simulink model "robot_controller"  (R2024a)
settings: Solver=FixedStepDiscrete  StartTime=0.0  StopTime=10.0  FixedStep=0.1  RelTol=1e-3  EnableMultiTasking=on
settings Model: ExtModeTrigDuration=2  Creator=amir  LastModifiedBy=amir
settings SolverCC: AutoInsertRateTranBlk=on  EnableFixedStepZeroCrossing=on
settings OptimizationCC: DefaultParameterBehavior=Inlined  UseDivisionForNetSlopeComputation=on  GainParamInheritBuiltInType=on  UseFloatMulNetSlope=on  InlineInvariantSignals=on  PassReuseOutputArgsAs=Individual arguments  ZeroExternalMemoryAtStartup=off  ZeroInternalMemoryAtStartup=off  NoFixptDivByZeroProtection=on  EfficientFloat2IntCast=on  LifeSpan=1  MaxStackSize=64  OptimizeBlockOrder=speed  DifferentSizesBufferReuse=on  EfficientTunableParamExpr=on
settings DebuggingCC: ParameterTunabilityLossMsg=error
settings HardwareCC: ProdBitPerInt=16  ProdBitPerPointer=16  ProdBitPerSizeT=16  ProdBitPerPtrDiffT=16  ProdLargestAtomicFloat=None  ProdWordSize=8  ProdLongLongMode=on  ProdHWDeviceType=Atmel->AVR
settings SFSimCC: MATLABDynamicMemAlloc=off
settings RTWCC: Description=Embedded Coder  SystemTargetFile=ert.tlc  HardwareBoard=Arduino Uno  TemplateMakefile=ert_default_tmf  Toolchain=Arduino AVR  BuildConfiguration=Faster Runs
settings CodeAppCC: ForceParamTrailComments=on  IgnoreCustomStorageClasses=off  OperatorAnnotations=on  SimulinkDataObjDesc=on  SFDataObjDesc=on  CustomSymbolStrGlobalVar=rt$N$M  CustomSymbolStrType=$N$M  CustomSymbolStrFcn=$N$M$F  CustomSymbolStrMacro=$N$M  InsertBlockDesc=on
settings ERTTargetCC: IncludeMdlTerminateFcn=off  CombineSignalStateStructs=on  SupportAbsoluteTime=off  SupportComplex=off  SupportNonInlinedSFcns=on  ExtModeTransport=3  ExtModeStaticAlloc=on  ExtModeAutomaticAllocSize=off  ExtModeStaticAllocSize=250  ExtModeMexFile=ext_xcp  ExtModeIntrfLevel=Level2 - Open  InlinedParameterPlacement=NonHierarchical  ERTFilePackagingFormat=CompactWithDataFile

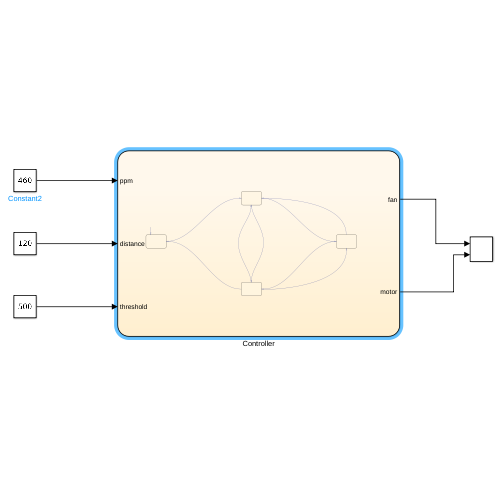
[thumbnail: Simulink's stored preview of the top-level diagram]
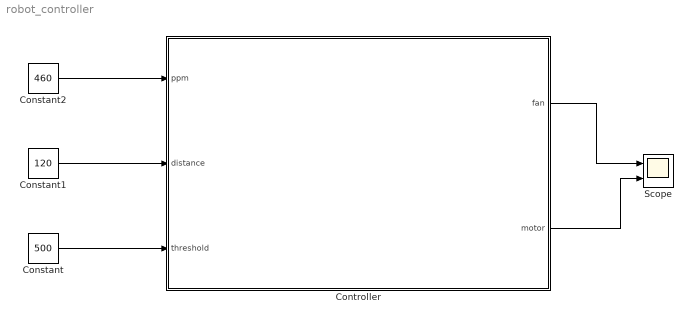
== system robot_controller ==
  Constant : Constant  Value=500
  Constant1 : Constant  Value=120
  Constant2 : Constant  Value=460
  Controller : Stateflow chart  TreatAsAtomicUnit=on
  Scope : Scope  NumInputPorts=2
  wires:
  Controller/1(fan) -> Scope/1
  Controller/2(motor) -> Scope/2
  Constant/1 -> Controller/3(threshold)
  Constant1/1 -> Controller/2(distance)
  Constant2/1 -> Controller/1(ppm)

== stateflow chart robot_controller/Controller ==
  state approach
  state idle
  state stay
  state retreat
  idle -> approach : [ppm > 400]{fan = 1; motor = 1;}
  stay -> approach [order 2] : [(ppm < threshold) & (distance > 110)]{motor = 1;}
  approach -> stay [order 2] : [(ppm < threshold) & (distance > 100 & distance < 110)]{motor = 0;}
  retreat -> approach [order 2] : [(ppm < threshold) & (distance > 110)]{fan = 1; motor = 1;}
  approach -> retreat [order 1] : [(ppm <= 400) | (ppm >= threshold) | (distance < 100)]{fan = 0; motor = -1;}
  (default) -> idle
  retreat -> idle [order 1] : [ppm <= 400]{fan = 0; motor = 0;}
  stay -> retreat [order 1] : [(ppm <= 400) | (ppm >= threshold) | (distance < 100)]{fan = 0; motor = -1;}
  retreat -> stay [order 3] : [(ppm < threshold) & (distance > 100 & distance < 110)]{motor = 0;}
  data: ppm input; distance input; threshold input; fan output; motor output
